simulink model "SalidaClase_Obstaculos"  (R2023b)
settings: Solver=FixedStepAuto  StartTime=0.0  StopTime=70  RelTol=1e-3  EnableMultiTasking=on
model workspace (MAT data in the model file):
  d = 0.15
libraries: SignalEditorBlockLib x2, robotalgslib x1
settings Model: ExtModeTrigDuration=2  Creator=Usuario  LastModifiedBy=Usuario
settings OptimizationCC: EnhancedBackFolding=on  PassReuseOutputArgsAs=Individual arguments  ZeroExternalMemoryAtStartup=off  ZeroInternalMemoryAtStartup=off  MaxStackSize=64  OptimizeBlockOrder=speed  DifferentSizesBufferReuse=on  OptimizationCustomize=off  EfficientTunableParamExpr=on
settings DebuggingCC: ParameterTunabilityLossMsg=error
settings HardwareCC: ProdBitPerInt=16  ProdBitPerPointer=16  ProdBitPerSizeT=16  ProdBitPerPtrDiffT=16  ProdLargestAtomicFloat=None  ProdWordSize=8  ProdHWDeviceType=Atmel->AVR  UseEmbeddedCoderFeatures=off  UseSimulinkCoderFeatures=off
settings SFSimCC: MATLABDynamicMemAlloc=off
settings RTWCC: Description=Embedded Coder  SystemTargetFile=ert.tlc  HardwareBoard=Arduino Mega 2560  TemplateMakefile=ert_default_tmf  Toolchain=Arduino AVR  BuildConfiguration=Faster Runs
settings CodeAppCC: ForceParamTrailComments=on  IgnoreCustomStorageClasses=off  OperatorAnnotations=on  SimulinkDataObjDesc=on  SFDataObjDesc=on  InsertBlockDesc=on
settings ERTTargetCC: SupportContinuousTime=on  SupportNonInlinedSFcns=on  SupportVariableSizeSignals=on  ExtModeTransport=3  ExtModeStaticAlloc=on  ExtModeAutomaticAllocSize=off  ExtModeStaticAllocSize=2048  ExtModeMexFile=ext_xcp  ExtModeIntrfLevel=Level2 - Open

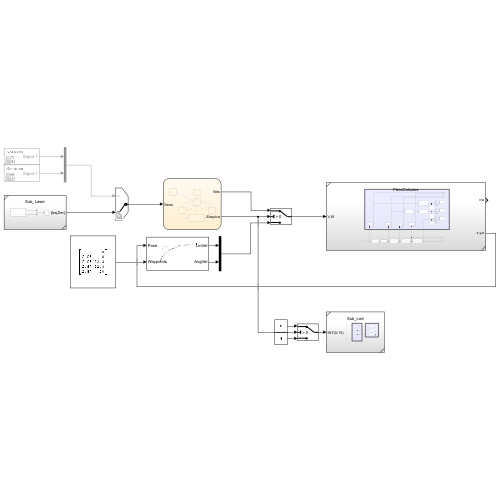
[thumbnail: Simulink's stored preview of the top-level diagram]
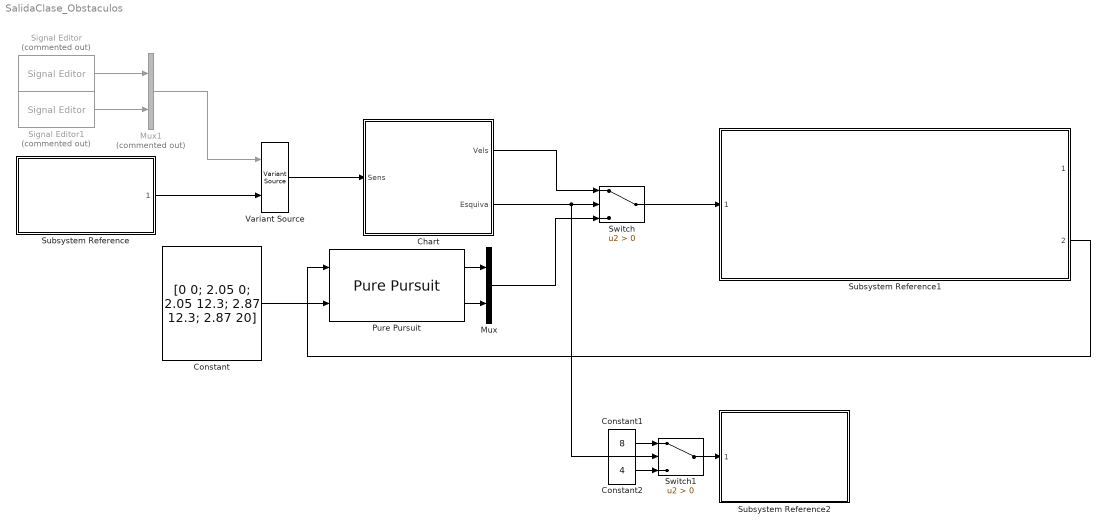
== system SalidaClase_Obstaculos ==
  Chart : Stateflow chart  TreatAsAtomicUnit=on
  Constant : Constant  Value=[0 0; 2.05 0; 2.05 12.3; 2.87 12.3; 2.87 20]
  Constant1 : Constant  Value=8
  Constant2 : Constant  Value=4
  Mux : Mux  Inputs=2
  Mux1 : Mux  Commented=on  Inputs=2
  Pure Pursuit : robotalgslib/Pure Pursuit  DesiredLinearVelocity=0.3  MaxAngularVelocity=pi/4  LookaheadDistance=0.5  TargetDirPort=off  SimulateUsing=Code generation
      settings: LibrarySourceBlock=robotmobilelib/Pure Pursuit
  Signal Editor : SignalEditorBlockLib/Signal Editor  Commented=on  FileName=Control10_SensorIzq.mat  ActiveScenario=Scenario  ActiveSignal=Signal 1  IsBus=off  OutputBusObjectStr=Bus: BusObject  SampleTime=0  Interpolate=off  ZeroCross=off  OutputAfterFinalValue=Setting to zero  Unit=inherit  PreserveSignalName=on  ApplySigPropsToAllScenarios=on  ApplySigPropsToAllSignals=off
  Signal Editor1 : SignalEditorBlockLib/Signal Editor  Commented=on  FileName=Control10_SensorDer.mat  ActiveScenario=Scenario  ActiveSignal=Signal 1  IsBus=off  OutputBusObjectStr=Bus: BusObject  SampleTime=0  Interpolate=off  ZeroCross=off  OutputAfterFinalValue=Setting to zero  Unit=inherit  PreserveSignalName=on  ApplySigPropsToAllScenarios=on  ApplySigPropsToAllSignals=off
  Subsystem Reference : Subsystem  ReferencedSubsystem=Sub_Laser
  Subsystem Reference1 : Subsystem  ReferencedSubsystem=PieroCalculos
  Subsystem Reference2 : Subsystem  ReferencedSubsystem=Sub_Led
  Switch : Switch  Criteria=u2 > Threshold  SaturateOnIntegerOverflow=off  InputSameDT=off
  Switch1 : Switch  Criteria=u2 > Threshold  SaturateOnIntegerOverflow=off  InputSameDT=off
  Variant Source : VariantSource  VariantControlMode=sim codegen switching
  wires:
  Switch/1 -> Subsystem Reference1/1
  Constant/1 -> Pure Pursuit/2
  Subsystem Reference1/2 -> Pure Pursuit/1
  Chart/1(Vels) -> Switch/1
  Pure Pursuit/2 -> Mux/2
  Pure Pursuit/1 -> Mux/1
  Mux/1 -> Switch/3
  Switch1/1 -> Subsystem Reference2/1
  Constant2/1 -> Switch1/3
  Constant1/1 -> Switch1/1
  Chart/2(Esquiva) -> Switch1/2, Switch/2
  Variant Source/1 -> Chart/1(Sens)
  Subsystem Reference/1 -> Variant Source/2
  Signal Editor1/1 -> Mux1/2
  Signal Editor/1 -> Mux1/1
  Mux1/1 -> Variant Source/1

== stateflow chart SalidaClase_Obstaculos/Chart ==
  settings: updateMethod=DISCRETE  sampleTime=0.01
  state Fin
    entry:
    Esquiva=1;
    Vels(1)=0;
    Vels(2)=0;
  state Inicio
    entry:
    Esquiva=0;
    Vels(1)=0;
    Vels(2)=0;
  state SinObstaculos
    entry:
    Esquiva=0;
    Vels(1)=0;
    Vels(2)=0;
  state Obst_Izq
    entry:
    Esquiva=1;
    Vels(1)=0.1;
    Vels(2)=-pi/3;
  state Obst_Der
    entry:
    Esquiva=1;
    Vels(1)=0.1;
    Vels(2)=+pi/3;
  state Obst_Enfrente
    entry:
    Esquiva=1;
    Vels(1)=0;
    Vels(2)=+pi/4*sign(Sens(1)-Sens(2));
  (default) -> Inicio
  SinObstaculos -> Fin [order 3] : after(70,sec)
  Inicio -> SinObstaculos : [after(1,sec)]
  SinObstaculos -> Obst_Izq [order 1] : [Sens(1)<350]
  SinObstaculos -> Obst_Der [order 2] : [Sens(2)<350]
  Obst_Izq -> SinObstaculos [order 1] : [Sens(1)>450]
  Obst_Enfrente -> SinObstaculos : after(2,sec)
  Obst_Der -> SinObstaculos [order 1] : [Sens(2)>450]
  Obst_Izq -> Obst_Enfrente [order 2] : [Sens(2)<400]
  Obst_Der -> Obst_Enfrente [order 2] : [Sens(1)<400]
  data: Vels output double size=2; Sens input size=2; Esquiva output double size=1
